simulink model "OFDM"  (R2021a)
settings: Solver=VariableStepAuto  StartTime=0.0  StopTime=10.0  RelTol=1e-3
libraries: commofdm x2, commdigbbndam3 x2, commchan3 x1, commrandsrc3 x1, commsink2 x1, dspstat3 x1, dspmathops x1
settings Model: Creator=RISHI  LastModifiedBy=suksi

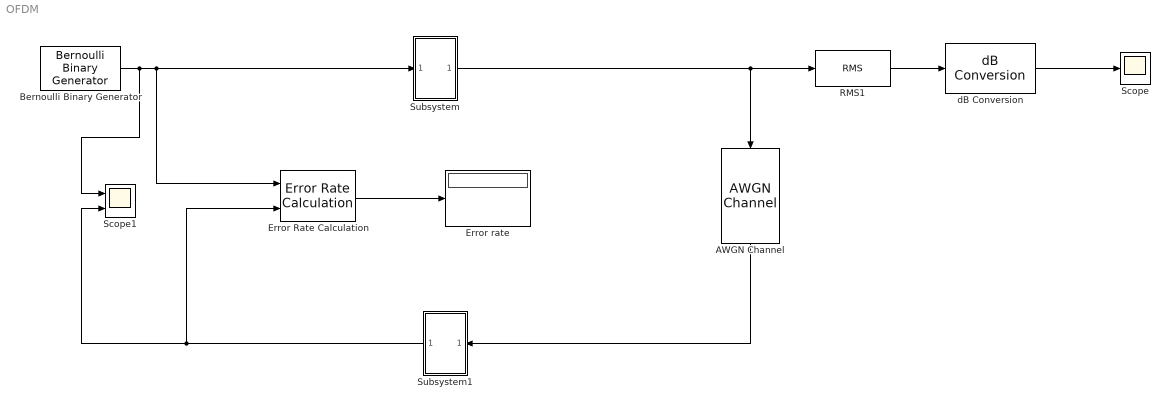
== system OFDM ==
  AWGN Channel : commchan3/AWGN Channel  InputProcessing=Columns as channels (frame based)  seed=67  noiseMode="Signal to noise ratio  (SNR)"  EbNodB=10  EsNodB=10  SNRdB=10  bitsPerSym=1  Ps=1  Tsym=1  variance=1
  Bernoulli Binary Generator : commrandsrc3/Bernoulli Binary Generator  ProbabilityOfZero=0.5  SeedSource=Auto  Seed=0  SampleTime=1/192  SamplesPerFrame=192  OutputDataType=boolean  SimulateUsing=Interpreted execution
  Error Rate Calculation : commsink2/Error Rate Calculation  N=0  st_delay=0  cp_mode=Entire frame  subframe=[]  PMode=Port  WsName=ErrorVec  RsMode2=off  stop=off  numErr=100  maxBits=1e6
  "Error rate " : Display
  RMS1 : dspstat3/RMS  run=off  directionMode=Each column  dimension=1  InputProcessing=Columns as channels (frame based)  reset_popup=None
  Scope : Scope
  Scope1 : Scope  NumInputPorts=2
  Subsystem : Subsystem  TreatAsAtomicUnit=on
  Subsystem1 : Subsystem
  dB Conversion : dspmathops/dB Conversion  dBtype=dB  intype=Amplitude  R=1  fuzz=off
  wires:
  Bernoulli Binary Generator/1 -> Scope1/1, Subsystem/1(In1), Error Rate Calculation/1
  Error Rate Calculation/1 -> "Error rate "/1
  dB Conversion/1 -> Scope/1
  RMS1/1 -> dB Conversion/1
  Subsystem/1(Out1) -> AWGN Channel/1, RMS1/1
  Subsystem1/1(Out1) -> Scope1/2, Error Rate Calculation/2
  AWGN Channel/1 -> Subsystem1/1(In1)

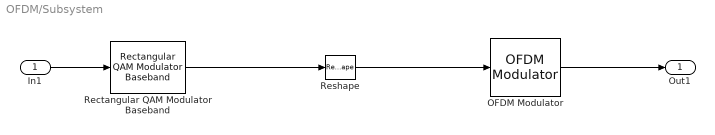
== system OFDM/Subsystem ==
  In1 : Inport
  OFDM Modulator : commofdm/OFDM Modulator  StatePerturbationForJacobian=1.0e-05  FFTLength=64  NumGuardBandCarriers=[8; 8]  InsertDCNull=off  PilotInputPort=off  PilotCarrierIndices=[12; 26; 40; 54]  CyclicPrefixLength=16  Windowing=off  WindowLength=1  NumSymbols=1  NumTransmitAntennas=1  SimulateUsing=Interpreted execution
      settings: SourceProductBaseCode=CM
  Rectangular QAM Modulator Baseband : commdigbbndam3/Rectangular QAM Modulator Baseband  M=16  InType=Bit  Enc=Gray  Mapping=[0:15]  PowType=Min. distance between symbols  MinDist=2  AvgPow=1  PeakPow=1  Ph=0  outDtype=double  outWordLen=16  outUDDataType=sfix(16)  outFracLenMode=Best precision  outFracLen=15  outDataTypeStr=double  outLastDataTypeStr=double
  Reshape : Reshape  OutputDimensionality=Customize  OutputDimensions=[48,1,1]
  Out1 : Outport
  wires:
  Rectangular QAM Modulator Baseband/1 -> Reshape/1
  Reshape/1 -> OFDM Modulator/1
  OFDM Modulator/1 -> Out1/1
  In1/1 -> Rectangular QAM Modulator Baseband/1

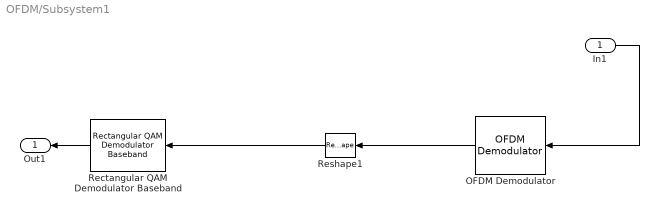
== system OFDM/Subsystem1 ==
  In1 : Inport
  OFDM Demodulator : commofdm/OFDM Demodulator  StatePerturbationForJacobian=1.0e-05  FFTLength=64  NumGuardBandCarriers=[8; 8]  RemoveDCCarrier=off  PilotOutputPort=off  PilotCarrierIndices=[12; 26; 40; 54]  CyclicPrefixLength=16  NumSymbols=1  NumReceiveAntennas=1  SimulateUsing=Interpreted execution
      settings: SourceProductBaseCode=CM
  Rectangular QAM Demodulator Baseband : commdigbbndam3/Rectangular QAM Demodulator Baseband  M=16  OutType=Bit  DecType=Hard decision  VarSource=Dialog  Variance=1  Dec=Gray  Mapping=[0:15]  PowType=Min. distance between symbols  MinDist=2  AvgPow=1  PeakPow=1  Ph=0  outDtype1=boolean  outDtype2=Inherit via internal rule  derotateFactorWordLen=16  derotateFactorDataTypeStr=Inherit: Same word length as input  derotateFactorLastDataTypeStr=Inherit: Same word length as input  denormFactorWordLen=16  denormFactorDataTypeStr=Inherit: Same word length as input  denormFactorLastDataTypeStr=Inherit: Same word length as input  prodOutWordLen=32  prodOutOverflowMode=Wrap  prodOutRoundingMode=Floor  prodOutOvFlMode=off  prodOutOvFlModeLastStrValue=off  sumWordLen=32
  Reshape1 : Reshape  OutputDimensionality=Customize  OutputDimensions=[48,1]
  Out1 : Outport
  wires:
  Reshape1/1 -> Rectangular QAM Demodulator Baseband/1
  OFDM Demodulator/1 -> Reshape1/1
  In1/1 -> OFDM Demodulator/1
  Rectangular QAM Demodulator Baseband/1 -> Out1/1
